simulink model "s17dot1_5filter"  (R2023b)
settings: Solver=FixedStepAuto  StartTime=0.0  StopTime=10.0  FixedStep=0.001  RelTol=1e-3
settings Model: Creator=lxj  LastModifiedBy=lxj
settings DataIOCC: LoadExternalInput=on
settings ConfigComp: CovScope=ReferencedModels

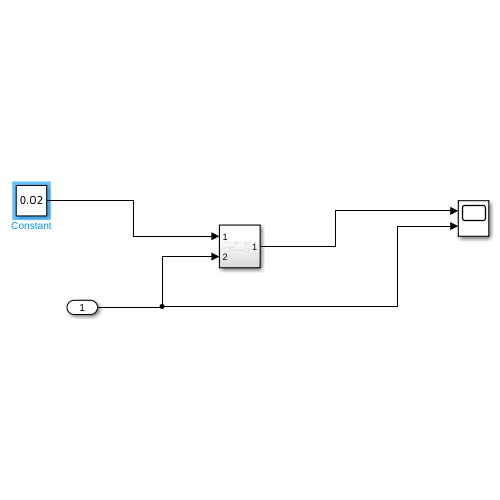
[thumbnail: Simulink's stored preview of the top-level diagram]
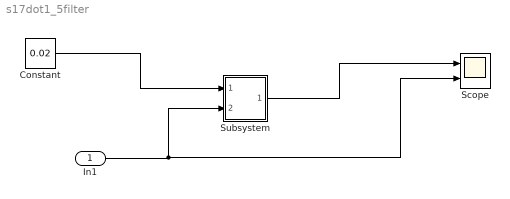
== system s17dot1_5filter ==
  In1 : Inport
  Constant : Constant  Value=0.02
  Scope : Scope  NumInputPorts=2
  Subsystem : Subsystem
  wires:
  Constant/1 -> Subsystem/1(In1)
  Subsystem/1(Out1) -> Scope/1
  In1/1 -> Scope/2, Subsystem/2(In2)

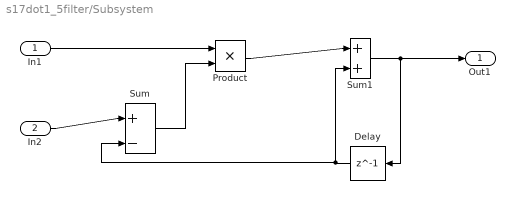
== system s17dot1_5filter/Subsystem ==
  In1 : Inport
  In2 : Inport  Port=2
  Delay : Delay  DelayLength=1  InitialCondition=0
  Product : Product
  Sum : Sum  Inputs=|+-
  Sum1 : Sum  Inputs=|++
  Out1 : Outport
  wires:
  In2/1 -> Sum/1
  In1/1 -> Product/1
  Delay/1 -> Sum/2, Sum1/2
  Sum/1 -> Product/2
  Product/1 -> Sum1/1
  Sum1/1 -> Out1/1, Delay/1
